simulink model "LandStation"  (R2023b)
settings: Solver=VariableStepAuto  StartTime=0.0  StopTime=10.0  RelTol=1e-3
settings Model: Creator=user  LastModifiedBy=user

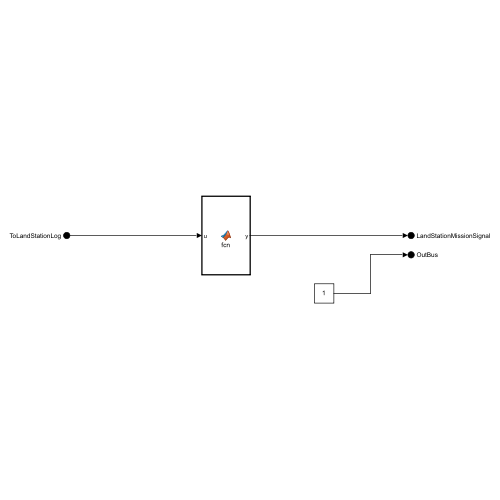
[thumbnail: Simulink's stored preview of the top-level diagram]
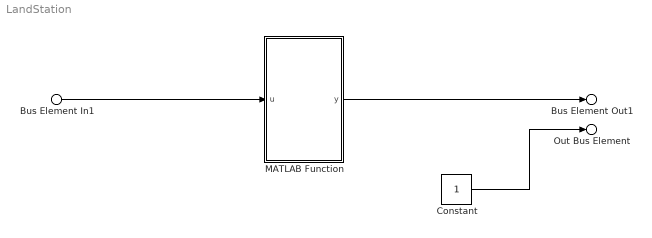
== system LandStation ==
  Bus Element In1 : Inport  PortName=ToLandStationLog
  Constant : Constant
  MATLAB Function : MATLAB Function  TreatAsAtomicUnit=on
  Bus Element Out1 : Outport  PortName=LandStationMissionSignal
  Out Bus Element : Outport  Port=2  PortName=OutBus
  wires:
  Bus Element In1/1 -> MATLAB Function/1(u)
  MATLAB Function/1(y) -> Bus Element Out1/1
  Constant/1 -> Out Bus Element/1

== matlab function LandStation/MATLAB Function ==
  data: u input; y output
function y = fcn(u)

MissionLog = u;

y = 1;
